simulink model "PTOSwt_DD"  (R2016b)
settings: configuration reference "CodeGenConfigSet" (kept outside this file)
values from neighbouring files (symbols this model uses):
  MoFPTO_uThresCalMsgA_CA = Calibration.Parameter    [init_PTOSwt_DD.m]
  MoFPTO_uTransf_CUR = Calibration.Parameter    [init_PTOSwt_DD.m]
  MoFPTO_uTransf_CURX = Calibration.Parameter    [init_PTOSwt_DD.m]
  PTOSwt_tiMaxDebDef_C = Calibration.Parameter    [init_PTOSwt_DD.m]
  PTOSwt_tiMaxDebOk_C = Calibration.Parameter    [init_PTOSwt_DD.m]
  PTOSwt_tiMinDebDef_C = Calibration.Parameter    [init_PTOSwt_DD.m]
  PTOSwt_tiMinDebOk_C = Calibration.Parameter    [init_PTOSwt_DD.m]
  PTOSwt_tiNplDebDef_C = Calibration.Parameter    [init_PTOSwt_DD.m]
  PTOSwt_tiNplDebOK_C = Calibration.Parameter    [init_PTOSwt_DD.m]
  PTOSwt_uSRCMax_C = Calibration.Parameter    [init_PTOSwt_DD.m]
  PTOSwt_uSRCMin_C = Calibration.Parameter    [init_PTOSwt_DD.m]
undefined symbols (not defined in the file or in its folder): PTOSwt_DD_DT
libraries: CXLib x9
settings Model: Creator=lenovo  LastModifiedBy=liutao
settings ConfigSetRef: SourceLocation=Base Workspace

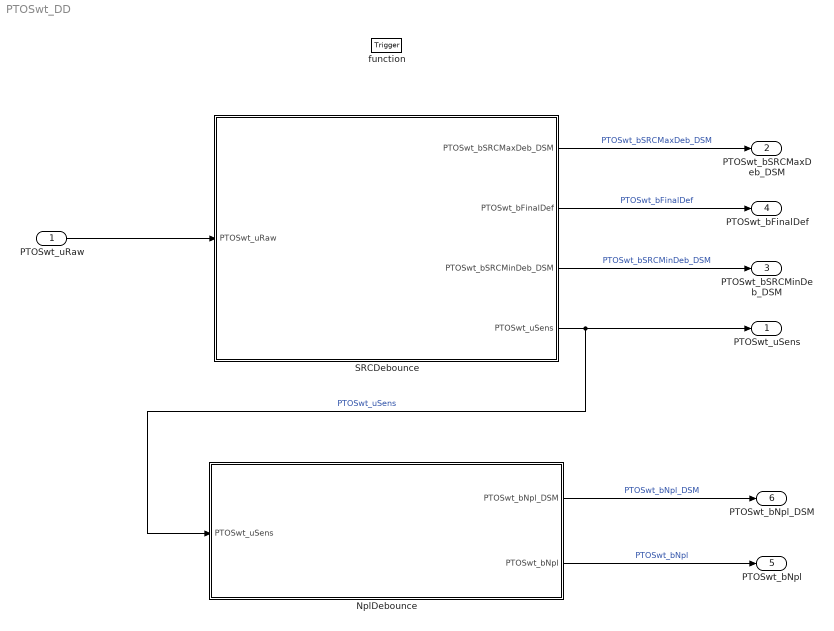
== system PTOSwt_DD ==
  PTOSwt_uRaw : Inport  Tag=mv  Description=Raw input voltage value for PTO switch  OutMin=0  OutMax=5000  OutDataTypeStr=Ad_mv
  function : TriggerPort  TriggerType=function-call  VariantControl=Variant
  NplDebounce : Subsystem
  SRCDebounce : Subsystem
  PTOSwt_uSens : Outport  Tag=mv  Description=Sensed value of multiple state switch  OutMin=0  OutMax=5000  OutDataTypeStr=Ad_mv
  PTOSwt_bSRCMaxDeb_DSM : Outport  Description="error state \"DFC_MaxPTOSwt\""  Port=2  OutMin=0  OutMax=1  OutDataTypeStr=boolean
  PTOSwt_bSRCMinDeb_DSM : Outport  Description="error state \"DFC_MinPTOSwt\""  Port=3  OutMin=0  OutMax=1  OutDataTypeStr=boolean
  PTOSwt_bFinalDef : Outport  Description=PTO switch sensor SRC finally defect flag  Port=4  OutMin=0  OutMax=1  OutDataTypeStr=boolean
  PTOSwt_bNpl : Outport  Description=PTO switch sensor non plausible flag  Port=5  OutMin=0  OutMax=1  OutDataTypeStr=boolean
  PTOSwt_bNpl_DSM : Outport  Description="error state \"DFC_NplPTOSwt\""  Port=6  OutMin=0  OutMax=1  OutDataTypeStr=boolean
  wires:
  SRCDebounce/4(PTOSwt_uSens) -> PTOSwt_uSens/1, NplDebounce/1(PTOSwt_uSens)  "PTOSwt_uSens"
  PTOSwt_uRaw/1 -> SRCDebounce/1(PTOSwt_uRaw)
  SRCDebounce/2(PTOSwt_bFinalDef) -> PTOSwt_bFinalDef/1  "PTOSwt_bFinalDef"
  NplDebounce/1(PTOSwt_bNpl_DSM) -> PTOSwt_bNpl_DSM/1  "PTOSwt_bNpl_DSM"
  NplDebounce/2(PTOSwt_bNpl) -> PTOSwt_bNpl/1  "PTOSwt_bNpl"
  SRCDebounce/3(PTOSwt_bSRCMinDeb_DSM) -> PTOSwt_bSRCMinDeb_DSM/1  "PTOSwt_bSRCMinDeb_DSM"
  SRCDebounce/1(PTOSwt_bSRCMaxDeb_DSM) -> PTOSwt_bSRCMaxDeb_DSM/1  "PTOSwt_bSRCMaxDeb_DSM"

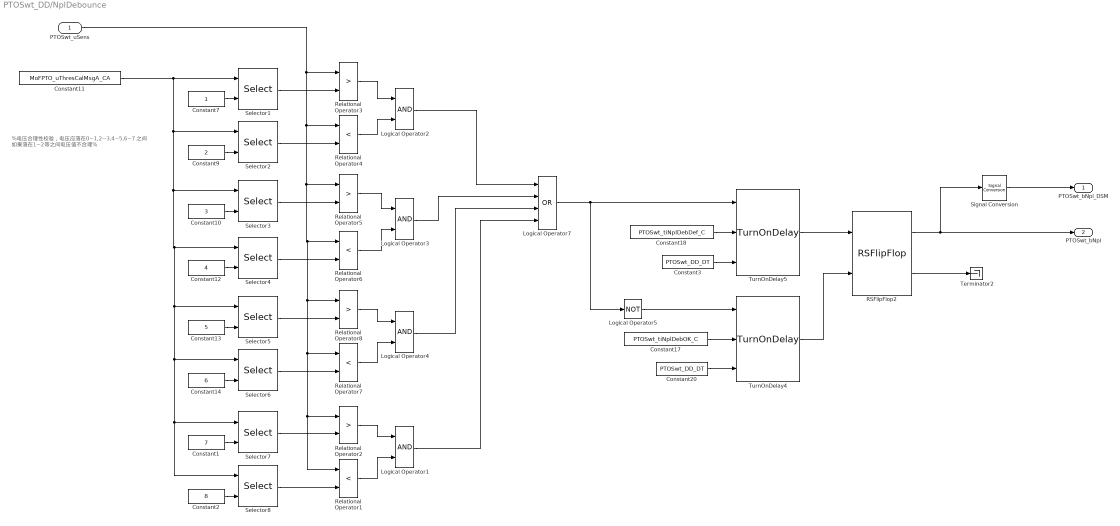
== system PTOSwt_DD/NplDebounce ==
  note: %电压合理性校验，电压应落在0~1,2~3,4~5,6~7之间
      | 如果落在1~2等之间电压值不合理%
  PTOSwt_uSens : Inport
  Constant1 : Constant  Value=7  OutDataTypeStr=uint8
  Constant10 : Constant  Value=3  OutDataTypeStr=uint8
  Constant11 : Constant  Value=MoFPTO_uThresCalMsgA_CA
  Constant12 : Constant  Value=4  OutDataTypeStr=uint8
  Constant13 : Constant  Value=5  OutDataTypeStr=uint8
  Constant14 : Constant  Value=6  OutDataTypeStr=uint8
  Constant17 : Constant  Value=PTOSwt_tiNplDebOK_C
  Constant18 : Constant  Value=PTOSwt_tiNplDebDef_C
  Constant2 : Constant  Value=8  OutDataTypeStr=uint8
  Constant20 : Constant  Value=PTOSwt_DD_DT  OutDataTypeStr=Inherit: Inherit via back propagation
  Constant3 : Constant  Value=PTOSwt_DD_DT  OutDataTypeStr=Inherit: Inherit via back propagation
  Constant7 : Constant  OutDataTypeStr=uint8
  Constant9 : Constant  Value=2  OutDataTypeStr=uint8
  Logical Operator{1..4} (4 alike) : Logic  AllPortsSameDT=off  OutDataTypeStr=boolean
  Logical Operator5 : Logic  Operator=NOT  AllPortsSameDT=off  OutDataTypeStr=boolean
  Logical Operator7 : Logic  Operator=OR  Inputs=4  AllPortsSameDT=off  OutDataTypeStr=boolean
  RSFlipFlop2 : CXLib/RSFlipFlop
  Relational Operator{1,4,6..7} (4 alike) : RelationalOperator  Operator=<  OutDataTypeStr=boolean  RndMeth=Nearest  InputSameDT=on
  Relational Operator{2..3,5,8} (4 alike) : RelationalOperator  Operator=>  OutDataTypeStr=boolean  RndMeth=Nearest  InputSameDT=on
  Selector{1..8} (8 alike) : Selector  IndexMode=Zero-based  InputPortWidth=10  IndexOptions=Index vector (port)  Indices=[1 3]  OutputSizes=1
  Signal Conversion : SignalConversion  OverrideOpt=off
  Terminator2 : Terminator
  TurnOnDelay4 : CXLib/TurnOnDelay
  TurnOnDelay5 : CXLib/TurnOnDelay
  PTOSwt_bNpl_DSM : Outport
  PTOSwt_bNpl : Outport  Port=2
  wires:
  Constant20/1 -> TurnOnDelay4/3
  TurnOnDelay5/1 -> RSFlipFlop2/1
  Constant3/1 -> TurnOnDelay5/3
  RSFlipFlop2/2 -> Terminator2/1
  Constant18/1 -> TurnOnDelay5/2
  Logical Operator5/1 -> TurnOnDelay4/1
  Constant17/1 -> TurnOnDelay4/2
  Logical Operator7/1 -> Logical Operator5/1, TurnOnDelay5/1
  TurnOnDelay4/1 -> RSFlipFlop2/2
  Constant14/1 -> Selector6/2
  Constant7/1 -> Selector1/2
  Relational Operator8/1 -> Logical Operator4/1
  Relational Operator4/1 -> Logical Operator2/2
  Relational Operator5/1 -> Logical Operator3/1
  Constant12/1 -> Selector4/2
  Constant9/1 -> Selector2/2
  Constant10/1 -> Selector3/2
  Constant13/1 -> Selector5/2
  Selector2/1 -> Relational Operator4/2
  Relational Operator3/1 -> Logical Operator2/1
  Selector1/1 -> Relational Operator3/2
  Relational Operator6/1 -> Logical Operator3/2
  Relational Operator7/1 -> Logical Operator4/2
  Selector5/1 -> Relational Operator8/2
  Selector3/1 -> Relational Operator5/2
  Selector4/1 -> Relational Operator6/2
  Selector6/1 -> Relational Operator7/2
  Logical Operator2/1 -> Logical Operator7/1
  Logical Operator3/1 -> Logical Operator7/2
  Logical Operator4/1 -> Logical Operator7/3
  RSFlipFlop2/1 -> PTOSwt_bNpl/1, Signal Conversion/1
  Signal Conversion/1 -> PTOSwt_bNpl_DSM/1
  PTOSwt_uSens/1 -> Relational Operator3/1, Relational Operator8/1, Relational Operator1/1, Relational Operator2/1, Relational Operator7/1, Relational Operator6/1, Relational Operator5/1, Relational Operator4/1
  Constant2/1 -> Selector8/2
  Relational Operator2/1 -> Logical Operator1/1
  Constant11/1 -> Selector2/1, Selector3/1, Selector4/1, Selector5/1, Selector6/1, Selector8/1, Selector7/1, Selector1/1
  Constant1/1 -> Selector7/2
  Relational Operator1/1 -> Logical Operator1/2
  Selector7/1 -> Relational Operator2/2
  Selector8/1 -> Relational Operator1/2
  Logical Operator1/1 -> Logical Operator7/4

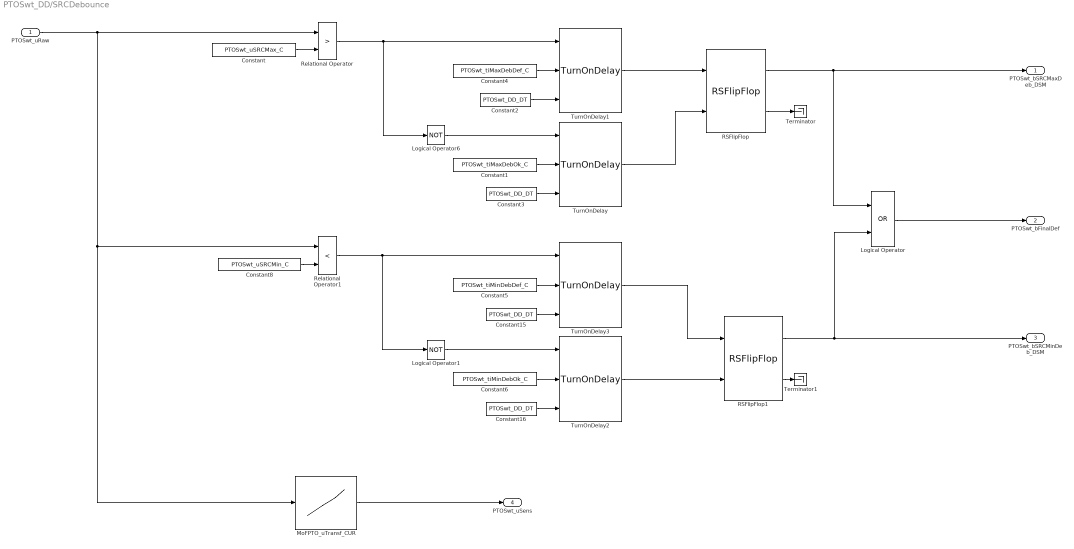
== system PTOSwt_DD/SRCDebounce ==
  PTOSwt_uRaw : Inport
  Constant : Constant  Value=PTOSwt_uSRCMax_C
  Constant1 : Constant  Value=PTOSwt_tiMaxDebOk_C
  Constant{2..3,15..16} (4 alike) : Constant  Value=PTOSwt_DD_DT  OutDataTypeStr=Inherit: Inherit via back propagation
  Constant4 : Constant  Value=PTOSwt_tiMaxDebDef_C
  Constant5 : Constant  Value=PTOSwt_tiMinDebDef_C
  Constant6 : Constant  Value=PTOSwt_tiMinDebOk_C
  Constant8 : Constant  Value=PTOSwt_uSRCMin_C
  Logical Operator : Logic  Operator=OR  AllPortsSameDT=off  OutDataTypeStr=boolean
  Logical Operator1 : Logic  Operator=NOT  AllPortsSameDT=off  OutDataTypeStr=boolean
  Logical Operator6 : Logic  Operator=NOT  AllPortsSameDT=off  OutDataTypeStr=boolean
  MoFPTO_uTransf_CUR : Lookup_n-D  NumberOfTableDimensions=1  BreakpointsForDimension1=MoFPTO_uTransf_CURX  IndexSearchMethod=Linear search  BeginIndexSearchUsingPreviousIndexResult=on  UseOneInputPortForAllInputData=on  Table=MoFPTO_uTransf_CUR  ExtrapMethod=Clip  UseLastTableValue=on  InternalRulePriority=Speed  OutDataTypeStr=Inherit: Inherit via back propagation  SaturateOnIntegerOverflow=on
  RSFlipFlop : CXLib/RSFlipFlop
  RSFlipFlop1 : CXLib/RSFlipFlop
  Relational Operator : RelationalOperator  Operator=>  OutDataTypeStr=boolean  RndMeth=Nearest  InputSameDT=on
  Relational Operator1 : RelationalOperator  Operator=<  OutDataTypeStr=boolean  RndMeth=Nearest  InputSameDT=on
  Terminator : Terminator
  Terminator1 : Terminator
  TurnOnDelay{,1..3} (4 alike) : CXLib/TurnOnDelay
  PTOSwt_bSRCMaxDeb_DSM : Outport
  PTOSwt_bFinalDef : Outport  Port=2
  PTOSwt_bSRCMinDeb_DSM : Outport  Port=3
  PTOSwt_uSens : Outport  Port=4
  wires:
  RSFlipFlop/1 -> PTOSwt_bSRCMaxDeb_DSM/1, Logical Operator/1
  RSFlipFlop1/1 -> PTOSwt_bSRCMinDeb_DSM/1, Logical Operator/2
  Constant/1 -> Relational Operator/2
  Constant8/1 -> Relational Operator1/2
  PTOSwt_uRaw/1 -> Relational Operator/1, MoFPTO_uTransf_CUR/1, Relational Operator1/1
  MoFPTO_uTransf_CUR/1 -> PTOSwt_uSens/1
  Logical Operator/1 -> PTOSwt_bFinalDef/1
  Logical Operator6/1 -> TurnOnDelay/1
  TurnOnDelay2/1 -> RSFlipFlop1/2
  Logical Operator1/1 -> TurnOnDelay2/1
  Constant1/1 -> TurnOnDelay/2
  TurnOnDelay/1 -> RSFlipFlop/2
  Relational Operator1/1 -> TurnOnDelay3/1, Logical Operator1/1
  TurnOnDelay1/1 -> RSFlipFlop/1
  Constant15/1 -> TurnOnDelay3/3
  RSFlipFlop/2 -> Terminator/1
  Constant5/1 -> TurnOnDelay3/2
  Constant16/1 -> TurnOnDelay2/3
  Constant4/1 -> TurnOnDelay1/2
  TurnOnDelay3/1 -> RSFlipFlop1/1
  Constant3/1 -> TurnOnDelay/3
  Constant6/1 -> TurnOnDelay2/2
  RSFlipFlop1/2 -> Terminator1/1
  Relational Operator/1 -> TurnOnDelay1/1, Logical Operator6/1
  Constant2/1 -> TurnOnDelay1/3
